simulink model "CruiseControlCarModel"  (R2021a)
settings: Solver=VariableStepAuto  StartTime=0.0  StopTime=10  RelTol=1e-3
StopFcn:
  | if (exist('SimulinkOutput', 'file')==2)
  | SimulinkOutput(out)
  | end
libraries: slpidlib x1
settings Model: Creator=vaibhavdeshmukh  LastModifiedBy=vdmac
settings SolverCC: AlgebraicLoopSolver=TrustRegion
settings DebuggingCC: SFMachineParentedDataDiag=warning

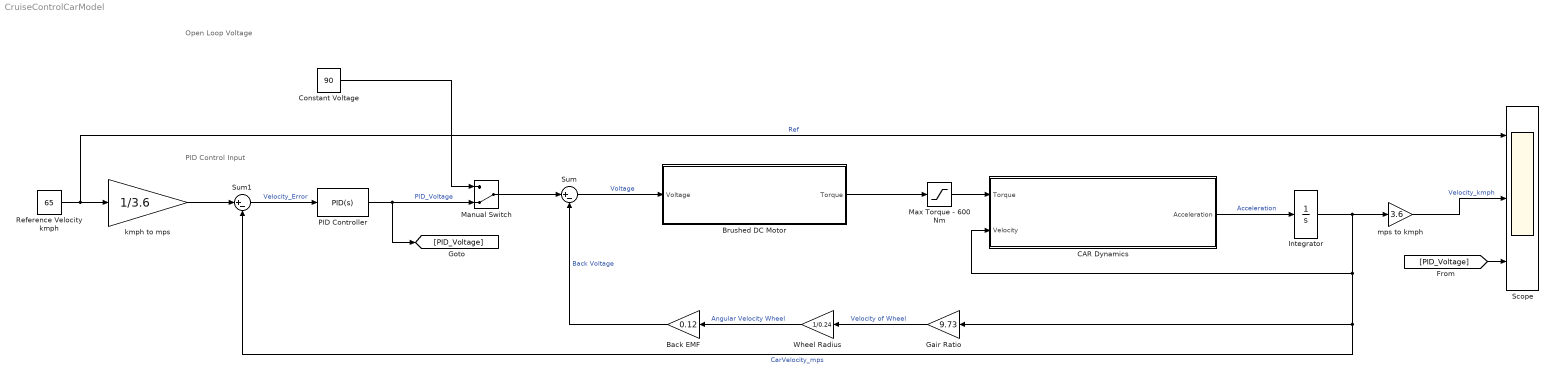
== system CruiseControlCarModel ==
  note: Open Loop Voltage
  note: PID Control Input
  Back EMF : Gain  Gain=0.12
  Brushed DC Motor : Subsystem
  CAR Dynamics : Subsystem
  Constant Voltage : Constant  Value=90
  Gair Ratio : Gain  Gain=9.73
  Integrator : Integrator
  Manual Switch : ManualSwitch  CurrentSetting=0
  Max Torque - 600 Nm : Saturate  UpperLimit=600  LowerLimit=0
  PID Controller : slpidlib/PID Controller  Controller=PID  Form=Parallel  TimeDomain=Continuous-time  UseExternalTs=off  SampleTime=-1  IntegratorMethod=Forward Euler  FilterMethod=Forward Euler  ControllerParametersSource=internal  P=200  I=10  D=15  UseFilter=on  N=100  TunerSelectOption=Transfer Function Based (PID Tuner App)  InitialConditionSource=internal  InitialConditionForIntegrator=0  InitialConditionForFilter=0  DifferentiatorICPrevScaledInput=0  ExternalReset=none  TrackingMode=off  Kt=1  LimitOutput=on  SatLimitsSource=internal  UpperSaturationLimit=346  LowerSaturationLimit=0  LinearizeAsGain=on  AntiWindupMode=none  Kb=1  POutMin=[]  POutMax=[]  IOutMin=[]  IOutMax=[]  DOutMin=[]  DOutMax=[]  NOutMin=[]  NOutMax=[]  SumOutMin=[]  SumOutMax=[]  SaturationOutMin=[]  SaturationOutMax=[]  PParamMin=[]  PParamMax=[]  IParamMin=[]  IParamMax=[]  DParamMin=[]  DParamMax=[]  NParamMin=[]  NParamMax=[]  KbParamMin=[]  KbParamMax=[]  KtParamMin=[]  KtParamMax=[]  KbOutMin=[]  KbOutMax=[]  KtOutMin=[]  KtOutMax=[]  IntegratorOutMin=[]  IntegratorOutMax=[]  FilterOutMin=[]  FilterOutMax=[]  SumI1OutMin=[]  SumI1OutMax=[]  SumI2OutMin=[]  SumI2OutMax=[]  SumI3OutMin=[]  SumI3OutMax=[]  SumI4OutMin=[]  SumI4OutMax=[]  SumDOutMin=[]  SumDOutMax=[]  DifferentiatorOutMin=[]  DifferentiatorOutMax=[]  FilterDiffOutCoefMin=[]  FilterDiffOutCoefMax=[]  ReciprocalOutMin=[]  ReciprocalOutMax=[]  SumDenOutMin=[]  SumDenOutMax=[]  SumNumOutMin=[]  SumNumOutMax=[]  DivideOutMin=[]  DivideOutMax=[]  UdiffTsProdOutMin=[]  UdiffTsProdOutMax=[]  NTsProdOutMin=[]  NTsProdOutMax=[]  UintegralTsProdOutMin=[]  UintegralTsProdOutMax=[]  UngainTsProdOutMin=[]  UngainTsProdOutMax=[]  IntegratorContinuousStateAttributes=''  IntegratorStateMustResolveToSignalObject=off  IntegratorRTWStateStorageClass=Auto  FilterContinuousStateAttributes=''  FilterStateMustResolveToSignalObject=off  FilterRTWStateStorageClass=Auto  ParallelPVariant=InternalParameters  IdealPVariant=Disabled  IVariant=InternalParameters  DVariant=InternalParameters  IntegratorVariant=Continuous  SatVariant=Enabled  AWVariant=Passthrough  PCopyVariant=Disabled  TRVariant=Disabled  FdbkBlocksVariant=Forward  IdealPFdbkVariant=Disabled  SatFdbkVariant=Disabled  DerivativeFilterVariant=ContFilter  NVariant=InternalParameters  NCopyVariant=Disabled  FilterICVariant=InternalICsFilter  IntegratorICVariant=InternalICs  ExternalResetVariant=Disabled  TRSumVariant=Passthrough  SumFdbkVariant=Disabled  SumVariant=Sum_PID  TsampFilterVariant=InternalTs  TsampNgainVariant=Passthrough  TsampIntegralVariant=Passthrough  ExternalSaturationOutDataTypeStr=Inherit: Same as second input
  Reference Velocity kmph : Constant  Value=65
  Scope : Scope  NumInputPorts=3
  Sum : Sum  Inputs=|+-
  Sum1 : Sum  Inputs=|+-
  Wheel Radius : Gain  Gain=1/0.24
  kmph to mps : Gain  Gain=1/3.6
  mps to kmph : Gain  Gain=3.6
  wires:
  CAR Dynamics/1(Acceleration) -> Integrator/1  "Acceleration"
  Integrator/1 -> Sum1/2, Gair Ratio/1, CAR Dynamics/2(Velocity), mps to kmph/1  "CarVelocity_mps"
  mps to kmph/1 -> Scope/2  "Velocity_kmph"
  Constant Voltage/1 -> Manual Switch/1
  Gair Ratio/1 -> Wheel Radius/1  "Velocity of Wheel"
  Wheel Radius/1 -> Back EMF/1  "Angular Velocity Wheel"
  Back EMF/1 -> Sum/2  "Back Voltage"
  Max Torque - 600 Nm/1 -> CAR Dynamics/1(Torque)
  Sum/1 -> Brushed DC Motor/1(Voltage)  "Voltage"
  Brushed DC Motor/1(Torque) -> Max Torque - 600 Nm/1
  kmph to mps/1 -> Sum1/1
  Reference Velocity kmph/1 -> Scope/1, kmph to mps/1  "Ref"
  Sum1/1 -> PID Controller/1  "Velocity_Error"
  PID Controller/1 -> [PID_Voltage], Manual Switch/2  "PID_Voltage"
  Manual Switch/1 -> Sum/1
  [PID_Voltage] -> Scope/3

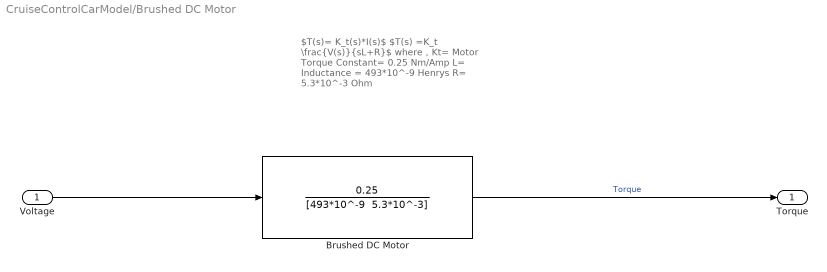
== system CruiseControlCarModel/Brushed DC Motor ==
  note: $T(s)= K_t(s)*I(s)$
      | $T(s) =K_t \frac{V(s)}{sL+R}$
      | where ,
      | Kt= Motor Torque Constant= 0.25 Nm/Amp
      | L= Inductance = 493*10^-9 Henrys
      | R= 5.3*10^-3 Ohm
  Voltage : Inport
  Brushed DC Motor : TransferFcn  Numerator=0.25  Denominator="[493*10^-9  5.3*10^-3]"
  Torque : Outport
  wires:
  Brushed DC Motor/1 -> Torque/1  "Torque"
  Voltage/1 -> Brushed DC Motor/1

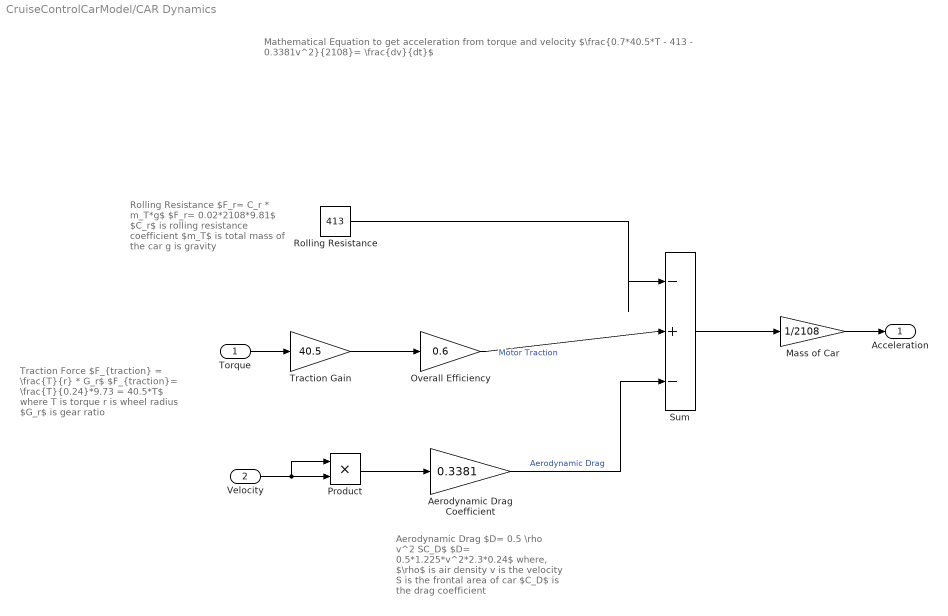
== system CruiseControlCarModel/CAR Dynamics ==
  note: Traction Force
      |
      | $F_{traction} = \frac{T}{r} * G_r$
      | $F_{traction}= \frac{T}{0.24}*9.73 = 40.5*T$
      | where
      | T is torque
      | r is wheel radius
      | $G_r$ is gear ratio
  note: Mathematical Equation to get acceleration from torque and velocity
      |
      | $\frac{0.7*40.5*T - 413 - 0.3381v^2}{2108}= \frac{dv}{dt}$
  note: Rolling Resistance
      | $F_r= C_r * m_T*g$
      | $F_r= 0.02*2108*9.81$
      |
      | $C_r$ is rolling resistance coefficient
      | $m_T$ is total mass of the car
      | g is gravity
  note: Aerodynamic Drag
      | $D= 0.5 \rho v^2 SC_D$
      | $D= 0.5*1.225*v^2*2.3*0.24$
      |
      | where,
      | $\rho$ is air density
      | v is the velocity
      | S is the frontal area of car
      | $C_D$ is the drag coefficient
  Torque : Inport
  Velocity : Inport  Port=2
  Aerodynamic Drag Coefficient : Gain  Gain=0.3381
  Mass of Car : Gain  Gain=1/2108
  Overall Efficiency : Gain  Gain=0.6
  Product : Product
  Rolling Resistance : Constant  Value=413
  Sum : Sum  Inputs=|-+-
  "Traction Gain " : Gain  Gain=40.5
  Acceleration : Outport
  wires:
  Torque/1 -> "Traction Gain "/1
  Velocity/1 -> Product/1, Product/2
  Aerodynamic Drag Coefficient/1 -> Sum/3  "Aerodynamic Drag"
  Overall Efficiency/1 -> Sum/2  "Motor Traction"
  Rolling Resistance/1 -> Sum/1
  Sum/1 -> Mass of Car/1
  Product/1 -> Aerodynamic Drag Coefficient/1
  Mass of Car/1 -> Acceleration/1
  "Traction Gain "/1 -> Overall Efficiency/1
